simulink model "px4demo_Read_Parameter"  (R2019b)
settings: Solver=FixedStepAuto  StartTime=0.0  StopTime=inf  RelTol=1e-3  EnableMultiTasking=on
libraries: px4lib x6, px4Sensorslib x1
settings Model: SimulationMode=external  ExtModeTrigDuration=10  Creator=The MathWorks, Inc.  LastModifiedBy=The MathWorks, Inc.
settings SolverCC: PositivePriorityOrder=on
settings DataIOCC: ReturnWorkspaceOutputs=off
settings OptimizationCC: EnhancedBackFolding=on  PassReuseOutputArgsAs=Individual arguments  ZeroExternalMemoryAtStartup=off  ZeroInternalMemoryAtStartup=off  MaxStackSize=64  OptimizeBlockOrder=speed  DifferentSizesBufferReuse=on  OptimizationCustomize=off  EfficientTunableParamExpr=on
settings DebuggingCC: ParameterTunabilityLossMsg=error  ArithmeticOperatorsInVariantConditions=warning
settings HardwareCC: ProdBitPerPointer=32  ProdBitPerSizeT=32  ProdBitPerPtrDiffT=32  ProdLargestAtomicInteger=Long  ProdLargestAtomicFloat=Double  ProdWordSize=32  ProdLongLongMode=on  ProdHWDeviceType=ARM Compatible->ARM Cortex
settings SFSimCC: MATLABDynamicMemAlloc=off
settings RTWCC: SystemTargetFile=ert.tlc  HardwareBoard=PX4 Pixhawk Series  TLCOptions="-aInlineSetEventsForThisBaseRateFcn=TLC_FALSE -aSuppressMultiTaskScheduler=TLC_FALSE    -aRateBasedStepFcn=0"  TemplateMakefile=ert_default_tmf  GenerateReport=on  Toolchain=GNU Tools for PX4 Autopilots  IncludeHyperlinkInReport=on  LaunchReport=on  TargetLang=C++  GenerateTraceInfo=on  GenerateTraceReport=on  GenerateTraceReportSl=on  GenerateTraceReportSf=on  GenerateTraceReportEml=on
settings CodeAppCC: ForceParamTrailComments=on  IgnoreCustomStorageClasses=off  OperatorAnnotations=on  SimulinkDataObjDesc=on  SFDataObjDesc=on  InsertBlockDesc=on
settings ERTTargetCC: ExtModeStaticAllocSize=2000

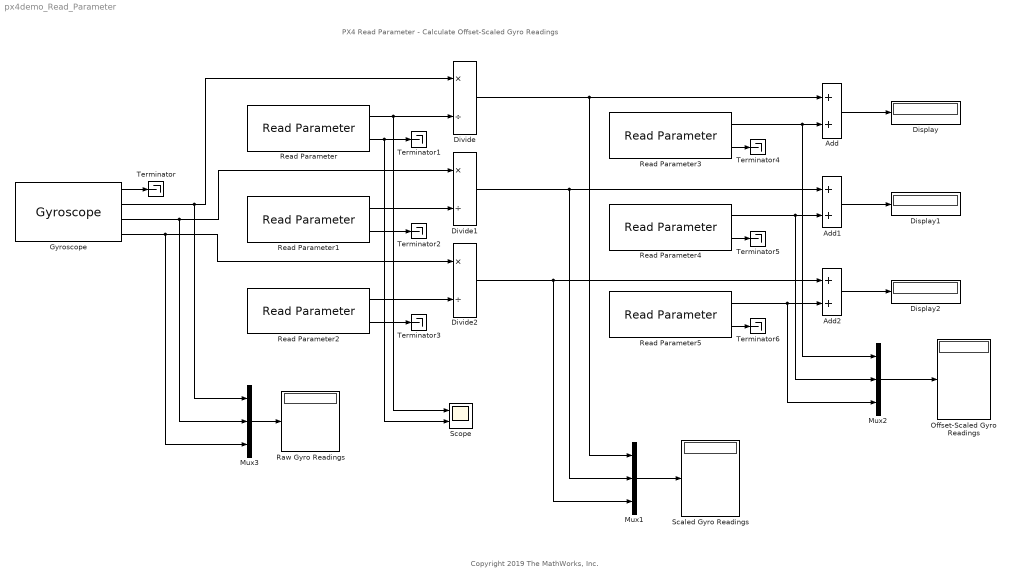
== system px4demo_Read_Parameter ==
  note: PX4 Read Parameter - Calculate Offset-Scaled Gyro Readings
  note: Copyright 2019 The MathWorks, Inc.
  Add : Sum
  Add1 : Sum
  Add2 : Sum
  Display : Display
  Display1 : Display
  Display2 : Display
  Divide : Product  Inputs=*/
  Divide1 : Product  Inputs=*/
  Divide2 : Product  Inputs=*/
  Gyroscope : px4Sensorslib/Gyroscope  uorbTimeStamp=off  BlockingMode=off  BlockTimeout=1e-3  sampleTime=1/250
      settings: SourceProductName=Embedded Coder Support Package for PX4 Autopilots  SourceProductBaseCode=PX4AUTOPILOTS
  Mux1 : Mux  Inputs=3
  Mux2 : Mux  Inputs=3
  Mux3 : Mux  Inputs=3
  Offset-Scaled Gyro Readings : Display
  Raw Gyro Readings : Display
  Read Parameter : px4lib/Read Parameter  ParameterName=CAL_GYRO0_XSCALE  DataType=FLOAT  SampleTime=inf
      settings: SourceProductName=Embedded Coder Support Package for PX4 Autopilots  SourceProductBaseCode=PX4AUTOPILOTS
  Read Parameter1 : px4lib/Read Parameter  ParameterName=CAL_GYRO0_YSCALE  DataType=FLOAT  SampleTime=inf
      settings: SourceProductName=Embedded Coder Support Package for PX4 Autopilots  SourceProductBaseCode=PX4AUTOPILOTS
  Read Parameter2 : px4lib/Read Parameter  ParameterName=CAL_GYRO0_ZSCALE  DataType=FLOAT  SampleTime=inf
      settings: SourceProductName=Embedded Coder Support Package for PX4 Autopilots  SourceProductBaseCode=PX4AUTOPILOTS
  Read Parameter3 : px4lib/Read Parameter  ParameterName=CAL_GYRO0_XOFF  DataType=FLOAT  SampleTime=inf
      settings: SourceProductName=Embedded Coder Support Package for PX4 Autopilots  SourceProductBaseCode=PX4AUTOPILOTS
  Read Parameter4 : px4lib/Read Parameter  ParameterName=CAL_GYRO0_YOFF  DataType=FLOAT  SampleTime=inf
      settings: SourceProductName=Embedded Coder Support Package for PX4 Autopilots  SourceProductBaseCode=PX4AUTOPILOTS
  Read Parameter5 : px4lib/Read Parameter  ParameterName=CAL_GYRO0_ZOFF  DataType=FLOAT  SampleTime=inf
      settings: SourceProductName=Embedded Coder Support Package for PX4 Autopilots  SourceProductBaseCode=PX4AUTOPILOTS
  Scaled Gyro Readings : Display
  Scope : Scope  NumInputPorts=2
  Terminator{,1..6} (7 alike) : Terminator
  wires:
  Gyroscope/2 -> Mux3/1, Divide/1
  Read Parameter2/1 -> Divide2/2
  Read Parameter5/1 -> Mux2/3, Add2/2
  Read Parameter1/1 -> Divide1/2
  Divide/1 -> Mux1/1, Add/1
  Divide1/1 -> Add1/1, Mux1/2
  Add2/1 -> Display2/1
  Mux1/1 -> Scaled Gyro Readings/1
  Divide2/1 -> Add2/1, Mux1/3
  Gyroscope/3 -> Mux3/2, Divide1/1
  Gyroscope/4 -> Mux3/3, Divide2/1
  Add/1 -> Display/1
  Read Parameter4/1 -> Mux2/2, Add1/2
  Read Parameter/1 -> Divide/2, Scope/1
  Mux2/1 -> Offset-Scaled Gyro Readings/1
  Read Parameter3/1 -> Mux2/1, Add/2
  Add1/1 -> Display1/1
  Gyroscope/1 -> Terminator/1
  Read Parameter/2 -> Scope/2, Terminator1/1
  Read Parameter1/2 -> Terminator2/1
  Read Parameter2/2 -> Terminator3/1
  Read Parameter3/2 -> Terminator4/1
  Read Parameter4/2 -> Terminator5/1
  Read Parameter5/2 -> Terminator6/1
  Mux3/1 -> Raw Gyro Readings/1
